simulink model "simulation"  (R2023b)
settings: Solver=ode1  StartTime=0.0  StopTime=90  FixedStep=0.01  RelTol=1e-3
undefined symbols (not defined in the file): A, B, C, dNx, dNy, dSx, dSy, g, kFD, kFT_N, kFT_S, Ki, kMD, kMDR_N, kMDR_S, Kx, m, w_hov, x0
libraries: SignalEditorBlockLib x1, shared6dof x1
settings Model: Creator=Rafa  LastModifiedBy=Rafa

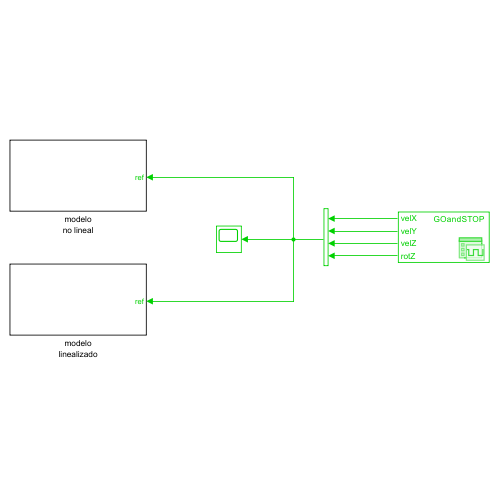
[thumbnail: Simulink's stored preview of the top-level diagram]
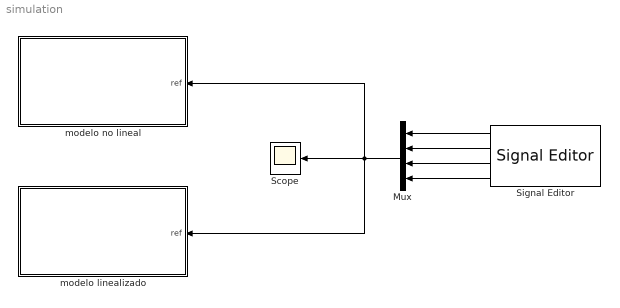
== system simulation ==
  Mux : Mux
  Scope : Scope
  Signal Editor : SignalEditorBlockLib/Signal Editor  FileName=C:\Users\Rafa\code\navsim\ws\src\navsim_pkg\models\UAM\aerotaxi\test\reference.mat  ActiveScenario=GOandSTOP  ActiveSignal=velX  IsBus=off  OutputBusObjectStr=Bus: BusObject  SampleTime=0  ZeroCross=off  OutputAfterFinalValue=Setting to zero  Unit=inherit  PreserveSignalName=on  ApplySigPropsToAllScenarios=on  ApplySigPropsToAllSignals=off
  modelo linealizado : Subsystem
      settings: PortSchema="{\"entries\":[{\"content\":{\"sides\":[{\"content\":{},\"type\":\"ConnectorPlacement.EquallySpacedRectSide\",\"uuid\":\"01253ba9-ebc4-4b01-a98e-e851f5719282\"},{\"content\":{\"connectorIds\":[\"In1\"],\"side\":\"RIGHT\"},\"type\":\"ConnectorPlacement.EquallySpacedRectSide\",\"uuid\":\"fb9dfd33-577f-4e16-aa58-2b7e19e1697c\"},{\"content\":{\"side\":\"TOP\"},\"type\":\"ConnectorPlacement.EquallySpacedRectSide\",\"uuid\":\"478e0daa-48f1-4d11-b0c5-5eb7f4b93804\"}]},\"type\":\"ConnectorPlacement.EquallySpacedConnector\",\"uuid\":\"8b8eac2c-ccef-432d-bf4d-f1cb8920e634\"}],\"packageUris\":[\"http://schema.mathworks.com/mf0/Connector/R2020b\"],\"version\":\"1.0\"}"
  modelo no lineal : Subsystem
      settings: PortSchema="{\"entries\":[{\"content\":{\"sides\":[{\"content\":{},\"type\":\"ConnectorPlacement.EquallySpacedRectSide\",\"uuid\":\"01253ba9-ebc4-4b01-a98e-e851f5719282\"},{\"content\":{\"connectorIds\":[\"In1\"],\"side\":\"RIGHT\"},\"type\":\"ConnectorPlacement.EquallySpacedRectSide\",\"uuid\":\"fb9dfd33-577f-4e16-aa58-2b7e19e1697c\"},{\"content\":{\"side\":\"TOP\"},\"type\":\"ConnectorPlacement.EquallySpacedRectSide\",\"uuid\":\"478e0daa-48f1-4d11-b0c5-5eb7f4b93804\"}]},\"type\":\"ConnectorPlacement.EquallySpacedConnector\",\"uuid\":\"8b8eac2c-ccef-432d-bf4d-f1cb8920e634\"}],\"packageUris\":[\"http://schema.mathworks.com/mf0/Connector/R2020b\"],\"version\":\"1.0\"}"
  wires:
  Signal Editor/4 -> Mux/4
  Signal Editor/2 -> Mux/2
  Signal Editor/1 -> Mux/1
  Signal Editor/3 -> Mux/3
  Mux/1 -> modelo linealizado/1(ref), modelo no lineal/1(ref), Scope/1

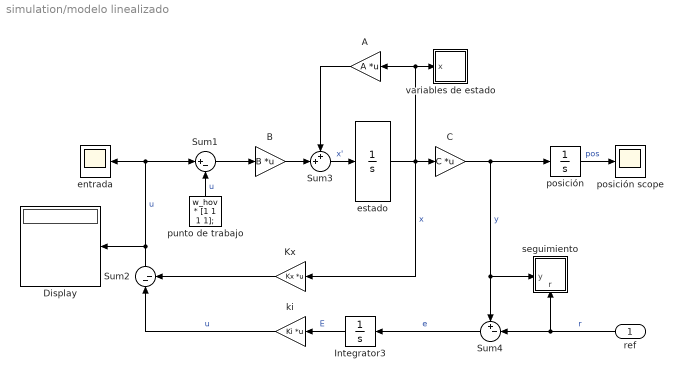
== system simulation/modelo linealizado ==
  ref : Inport
  A : Gain  Gain=A  Multiplication=Matrix(K*u)
  B : Gain  Gain=B  Multiplication=Matrix(K*u)
  C : Gain  Gain=C  Multiplication=Matrix(K*u)
  Display : Display
  Integrator3 : Integrator
  Kx : Gain  Gain=Kx  Multiplication=Matrix(K*u)
  Sum1 : Sum  Inputs=|+-
  Sum2 : Sum  Inputs=|--
  Sum3 : Sum  Inputs=++|
  Sum4 : Sum  Inputs=+-|
  entrada : Scope
  estado : Integrator  InitialCondition=x0
  ki : Gain  Gain=Ki  Multiplication=Matrix(K*u)
  posición : Integrator
  posición scope : Scope
  punto de trabajo : Constant  Value=w_hov * [1 1 1 1];
  seguimiento : Subsystem
      settings: PortSchema="{\"entries\":[{\"content\":{\"sides\":[{\"content\":{\"connectorIds\":[\"In1\"]},\"type\":\"ConnectorPlacement.EquallySpacedRectSide\",\"uuid\":\"d2eeeb7d-5f4a-4029-9315-eebcbcb452dd\"},{\"content\":{\"side\":\"RIGHT\"},\"type\":\"ConnectorPlacement.EquallySpacedRectSide\",\"uuid\":\"1640c7e1-69ae-41c3-aa10-8b2b7f223d3a\"},{\"content\":{\"side\":\"TOP\"},\"type\":\"ConnectorPlacement.EquallySpacedRectSide\",\"uuid\":\"4c9f5258-e874-4895-bd38-20065386e5c3\"},{\"content\":{\"connectorIds\":[\"In2\"],\"side\":\"BOTTOM\"},\"type\":\"ConnectorPlacement.EquallySpacedRectSide\",\"uuid\":\"545f1ef5-84f5-4856-98df-d523d3a0e9d2\"}]},\"type\":\"ConnectorPlacement.EquallySpacedConnector\",\"uuid\":\"43c46751-3b9a-4101-a1bf-f12efbef3486\"}],\"packageUris\":[\"http://schema.mathworks.com/mf0/Connector/R2020b\"],\"version\":\"1.0\"}"
  variables de estado : Subsystem
  wires:
  C/1 -> posición/1, Sum4/1, seguimiento/1(y)  "y"
  Sum1/1 -> B/1
  estado/1 -> Kx/1, A/1, variables de estado/1(x), C/1  "x"
  B/1 -> Sum3/2
  posición/1 -> posición scope/1  "pos"
  A/1 -> Sum3/1
  ref/1 -> seguimiento/2(r), Sum4/2  "r"
  ki/1 -> Sum2/1  "u"
  Sum4/1 -> Integrator3/1  "e"
  punto de trabajo/1 -> Sum1/2  "u"
  Sum2/1 -> Sum1/1, entrada/1, Display/1  "u"
  Sum3/1 -> estado/1  "x'"
  Kx/1 -> Sum2/2
  Integrator3/1 -> ki/1  "E"

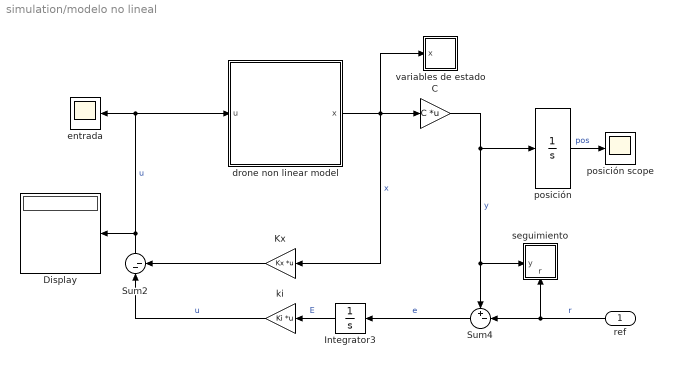
== system simulation/modelo no lineal ==
  ref : Inport
  C : Gain  Gain=C  Multiplication=Matrix(K*u)
  Display : Display
  Integrator3 : Integrator
  Kx : Gain  Gain=Kx  Multiplication=Matrix(K*u)
  Sum2 : Sum  Inputs=|--
  Sum4 : Sum  Inputs=+-|
  drone non linear model : Subsystem
  entrada : Scope
  ki : Gain  Gain=Ki  Multiplication=Matrix(K*u)
  posición : Integrator
  posición scope : Scope
  seguimiento : Subsystem
      settings: PortSchema="{\"entries\":[{\"content\":{\"sides\":[{\"content\":{\"connectorIds\":[\"In1\"]},\"type\":\"ConnectorPlacement.EquallySpacedRectSide\",\"uuid\":\"d2eeeb7d-5f4a-4029-9315-eebcbcb452dd\"},{\"content\":{\"side\":\"RIGHT\"},\"type\":\"ConnectorPlacement.EquallySpacedRectSide\",\"uuid\":\"1640c7e1-69ae-41c3-aa10-8b2b7f223d3a\"},{\"content\":{\"side\":\"TOP\"},\"type\":\"ConnectorPlacement.EquallySpacedRectSide\",\"uuid\":\"4c9f5258-e874-4895-bd38-20065386e5c3\"},{\"content\":{\"connectorIds\":[\"In2\"],\"side\":\"BOTTOM\"},\"type\":\"ConnectorPlacement.EquallySpacedRectSide\",\"uuid\":\"545f1ef5-84f5-4856-98df-d523d3a0e9d2\"}]},\"type\":\"ConnectorPlacement.EquallySpacedConnector\",\"uuid\":\"43c46751-3b9a-4101-a1bf-f12efbef3486\"}],\"packageUris\":[\"http://schema.mathworks.com/mf0/Connector/R2020b\"],\"version\":\"1.0\"}"
  variables de estado : Subsystem
  wires:
  Integrator3/1 -> ki/1  "E"
  Kx/1 -> Sum2/2
  Sum2/1 -> Display/1, drone non linear model/1(u), entrada/1  "u"
  Sum4/1 -> Integrator3/1  "e"
  ki/1 -> Sum2/1  "u"
  ref/1 -> Sum4/2, seguimiento/2(r)  "r"
  posición/1 -> posición scope/1  "pos"
  drone non linear model/1(x) -> C/1, variables de estado/1(x), Kx/1  "x"
  C/1 -> seguimiento/1(y), Sum4/1, posición/1  "y"

== system simulation/modelo linealizado/seguimiento ==
  y : Inport
  r : Inport  Port=2
  seguimiento de la referencia : Scope  NumInputPorts=2
  y Demux : Demux
  y Demux1 : Demux
  y Mux : Mux
  y Mux1 : Mux
  wires:
  y Demux/1 -> y Mux/1  "bXdot"
  y Demux/2 -> y Mux/2  "bYdot"
  y Demux/3 -> y Mux/3  "bZdot"
  y Mux/1 -> seguimiento de la referencia/1
  y Demux/4 -> y Mux/4  "bWz"
  y/1 -> y Demux/1
  r/1 -> y Demux1/1
  y Demux1/4 -> y Mux1/4  "bWz"
  y Mux1/1 -> seguimiento de la referencia/2
  y Demux1/3 -> y Mux1/3  "bZdot"
  y Demux1/2 -> y Mux1/2  "bYdot"
  y Demux1/1 -> y Mux1/1  "bXdot"

== system simulation/modelo linealizado/variables de estado ==
  x : Inport
  Demux : Demux  Outputs=8
  Mux : Mux  Inputs=8
  estado : Scope
  wires:
  Demux/6 -> Mux/6  "bXdot"
  Demux/7 -> Mux/7  "bYdot"
  Demux/8 -> Mux/8  "bZdot"
  Demux/2 -> Mux/2  "eTheta"
  Mux/1 -> estado/1
  Demux/4 -> Mux/4  "bWy"
  Demux/5 -> Mux/5  "bWz"
  Demux/1 -> Mux/1  "ePhi"
  Demux/3 -> Mux/3  "bWx"
  x/1 -> Demux/1

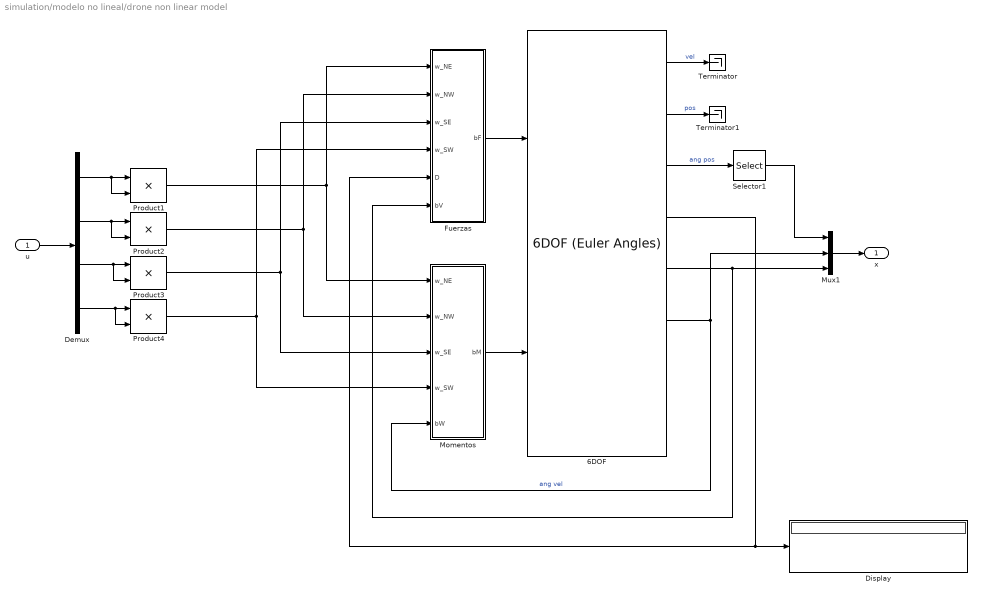
== system simulation/modelo no lineal/drone non linear model ==
  u : Inport
  6DOF : shared6dof/6DOF (Euler Angles)  units=Metric (MKS)  mtype=Fixed  rep=Euler Angles  xme_0=[0 0 0]  Vm_0=x0(6:8)  eul_0=[x0(1) x0(2) 0]  pm_0=x0(3:5)  mass_0=m  mass_e=0.5  mass_f=2.0  inertia=inertia  inertia_e=eye(3)  inertia_f=2*eye(3)  k_quat=1.0  vre_flag=on  abi_flag=off  aMode=aMode  xme_statename=''  Vm_statename=''  eul_statename=''  quat_statename=''  pm_statename=''  mass_statename=''
  Demux : Demux
  Display : Display
  Fuerzas : Subsystem
  Momentos : Subsystem
  Mux1 : Mux  Inputs=3
  Product{1..4} (4 alike) : Product
  Selector1 : Selector  InputPortWidth=3  IndexOptions=Index vector (dialog)  Indices=[1 2]  OutputSizes=1
  Terminator : Terminator
  Terminator1 : Terminator
  x : Outport  VectorParamsAs1DForOutWhenUnconnected=off
  wires:
  Product1/1 -> Fuerzas/1(w_NE), Momentos/1(w_NE)
  Product2/1 -> Fuerzas/2(w_NW), Momentos/2(w_NW)
  Product3/1 -> Fuerzas/3(w_SE), Momentos/3(w_SE)
  Product4/1 -> Fuerzas/4(w_SW), Momentos/4(w_SW)
  6DOF/4 -> Fuerzas/5(D), Display/1
  6DOF/6 -> Momentos/5(bW), Mux1/2  "ang vel"
  6DOF/5 -> Fuerzas/6(bV), Mux1/3
  6DOF/1 -> Terminator/1  "vel"
  6DOF/2 -> Terminator1/1  "pos"
  6DOF/3 -> Selector1/1  "ang pos"
  Mux1/1 -> x/1
  Selector1/1 -> Mux1/1
  u/1 -> Demux/1
  Fuerzas/1(bF) -> 6DOF/1
  Momentos/1(bM) -> 6DOF/2
  Demux/1 -> Product1/2, Product1/1
  Demux/2 -> Product2/2, Product2/1
  Demux/4 -> Product4/2, Product4/1
  Demux/3 -> Product3/2, Product3/1

== system simulation/modelo no lineal/seguimiento ==
  y : Inport
  r : Inport  Port=2
  seguimiento de la referencia : Scope  NumInputPorts=2
  y Demux : Demux
  y Demux1 : Demux
  y Mux : Mux
  y Mux1 : Mux
  wires:
  y Demux1/1 -> y Mux1/1  "bXdot"
  y Demux1/2 -> y Mux1/2  "bYdot"
  y Demux1/3 -> y Mux1/3  "bZdot"
  y Mux1/1 -> seguimiento de la referencia/2
  y Demux1/4 -> y Mux1/4  "bWz"
  r/1 -> y Demux1/1
  y/1 -> y Demux/1
  y Demux/4 -> y Mux/4  "bWz"
  y Mux/1 -> seguimiento de la referencia/1
  y Demux/3 -> y Mux/3  "bZdot"
  y Demux/2 -> y Mux/2  "bYdot"
  y Demux/1 -> y Mux/1  "bXdot"

== system simulation/modelo no lineal/variables de estado ==
  x : Inport
  Demux : Demux  Outputs=8
  Mux : Mux  Inputs=8
  estado : Scope
  wires:
  x/1 -> Demux/1
  Demux/3 -> Mux/3  "bWx"
  Demux/1 -> Mux/1  "ePhi"
  Demux/5 -> Mux/5  "bWz"
  Demux/4 -> Mux/4  "bWy"
  Mux/1 -> estado/1
  Demux/2 -> Mux/2  "eTheta"
  Demux/8 -> Mux/8  "bZdot"
  Demux/7 -> Mux/7  "bYdot"
  Demux/6 -> Mux/6  "bXdot"

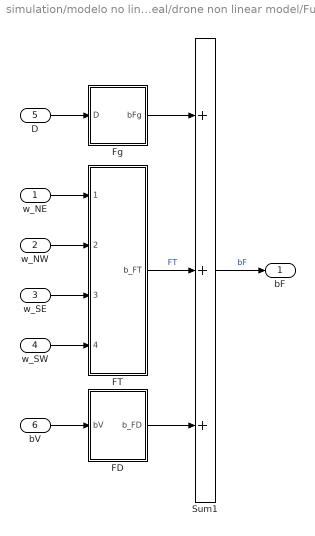
== system simulation/modelo no lineal/drone non linear model/Fuerzas ==
  w_NE : Inport
  w_NW : Inport  Port=2
  w_SE : Inport  Port=3
  w_SW : Inport  Port=4
  D : Inport  Port=5
  bV : Inport  Port=6
  FD : Subsystem
  FT : Subsystem
  Fg : Subsystem
  Sum1 : Sum  Inputs=+++
  bF : Outport  VectorParamsAs1DForOutWhenUnconnected=off
  wires:
  D/1 -> Fg/1(D)
  Fg/1(bFg) -> Sum1/1
  FT/1(b_FT) -> Sum1/2  "FT"
  w_SW/1 -> FT/4(w_SW)
  w_NE/1 -> FT/1(w_NE)
  w_SE/1 -> FT/3(w_SE)
  w_NW/1 -> FT/2(w_NW)
  Sum1/1 -> bF/1  "bF"
  bV/1 -> FD/1(bV)
  FD/1(b_FD) -> Sum1/3

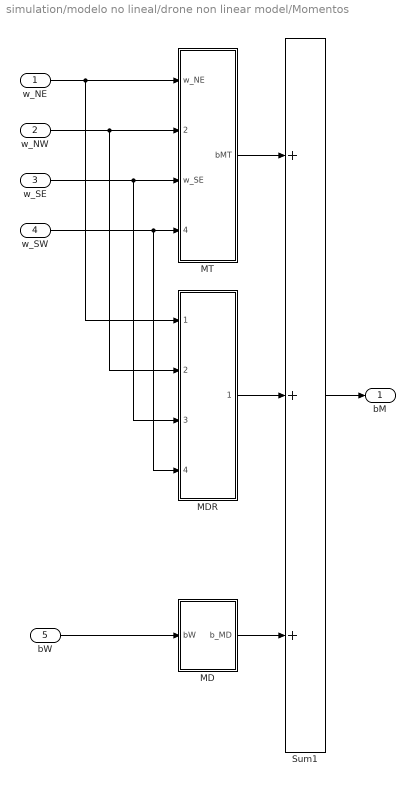
== system simulation/modelo no lineal/drone non linear model/Momentos ==
  w_NE : Inport
  w_NW : Inport  Port=2
  w_SE : Inport  Port=3
  w_SW : Inport  Port=4
  bW : Inport  Port=5
  MD : Subsystem
  MDR : Subsystem
  MT : Subsystem
  Sum1 : Sum  Inputs=+++
  bM : Outport  VectorParamsAs1DForOutWhenUnconnected=off
  wires:
  bW/1 -> MD/1(bW)
  MT/1(bMT) -> Sum1/1
  w_SW/1 -> MDR/4(w_SW), MT/4(w_SW)
  w_NE/1 -> MDR/1(w_NE), MT/1(w_NE)
  w_SE/1 -> MDR/3(w_SE), MT/3(w_SE)
  w_NW/1 -> MDR/2(w_NW), MT/2(w_NW)
  Sum1/1 -> bM/1
  MD/1(b_MD) -> Sum1/3
  MDR/1(b_MDR) -> Sum1/2

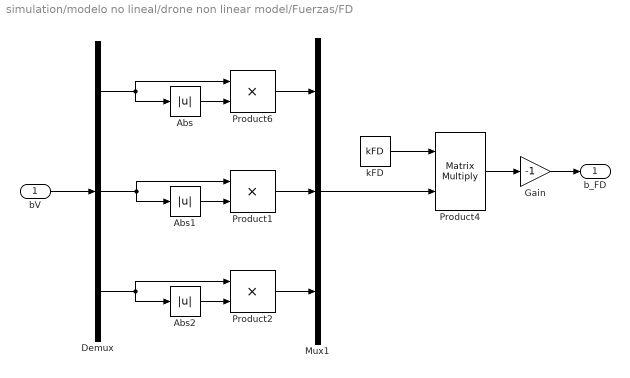
== system simulation/modelo no lineal/drone non linear model/Fuerzas/FD ==
  bV : Inport
  Abs : Abs  SaturateOnIntegerOverflow=off
  Abs1 : Abs  SaturateOnIntegerOverflow=off
  Abs2 : Abs  SaturateOnIntegerOverflow=off
  Demux : Demux  Outputs=3
  Gain : Gain  Gain=-1
  Mux1 : Mux  Inputs=3
  Product1 : Product
  Product2 : Product
  Product4 : Product  Multiplication=Matrix(*)
  Product6 : Product
  kFD : Constant  Value=kFD
  b_FD : Outport  VectorParamsAs1DForOutWhenUnconnected=off
  wires:
  kFD/1 -> Product4/1
  Product4/1 -> Gain/1
  Mux1/1 -> Product4/2
  Product1/1 -> Mux1/2
  bV/1 -> Demux/1
  Abs/1 -> Product6/2
  Abs1/1 -> Product1/2
  Abs2/1 -> Product2/2
  Demux/1 -> Product6/1, Abs/1
  Demux/2 -> Product1/1, Abs1/1
  Demux/3 -> Product2/1, Abs2/1
  Product6/1 -> Mux1/1
  Product2/1 -> Mux1/3
  Gain/1 -> b_FD/1

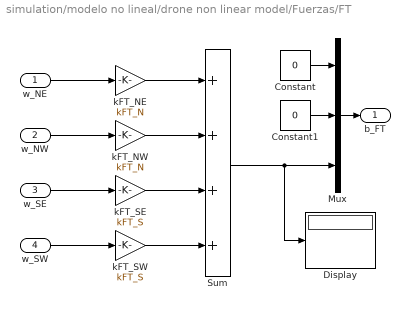
== system simulation/modelo no lineal/drone non linear model/Fuerzas/FT ==
  w_NE : Inport
  w_NW : Inport  Port=2
  w_SE : Inport  Port=3
  w_SW : Inport  Port=4
  Constant : Constant  Value=0
  Constant1 : Constant  Value=0
  Display : Display
  Mux : Mux  Inputs=3
  Sum : Sum  Inputs=++++
  kFT_NE : Gain  Gain=kFT_N
  kFT_NW : Gain  Gain=kFT_N
  kFT_SE : Gain  Gain=kFT_S
  kFT_SW : Gain  Gain=kFT_S
  b_FT : Outport  VectorParamsAs1DForOutWhenUnconnected=off
  wires:
  Mux/1 -> b_FT/1
  Constant/1 -> Mux/1
  Constant1/1 -> Mux/2
  Sum/1 -> Display/1, Mux/3
  w_NE/1 -> kFT_NE/1
  w_NW/1 -> kFT_NW/1
  w_SE/1 -> kFT_SE/1
  w_SW/1 -> kFT_SW/1
  kFT_NW/1 -> Sum/2
  kFT_NE/1 -> Sum/1
  kFT_SW/1 -> Sum/4
  kFT_SE/1 -> Sum/3

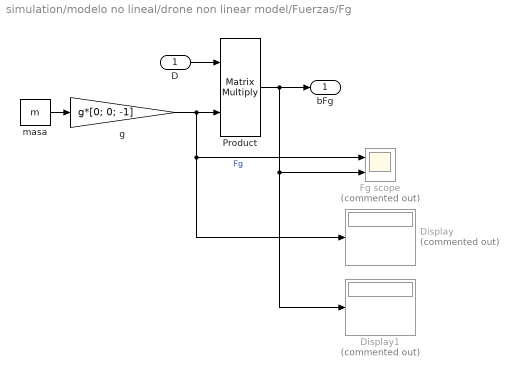
== system simulation/modelo no lineal/drone non linear model/Fuerzas/Fg ==
  D : Inport
  Display : Display  Commented=on
  Display1 : Display  Commented=on
  Fg scope : Scope  Commented=on  NumInputPorts=2
  Product : Product  Multiplication=Matrix(*)
  g : Gain  Gain=g*[0; 0; -1]
  masa : Constant  Value=m
  bFg : Outport  VectorParamsAs1DForOutWhenUnconnected=off
  wires:
  Product/1 -> Display1/1, Fg scope/2, bFg/1
  D/1 -> Product/1
  masa/1 -> g/1
  g/1 -> Display/1, Fg scope/1, Product/2  "Fg"

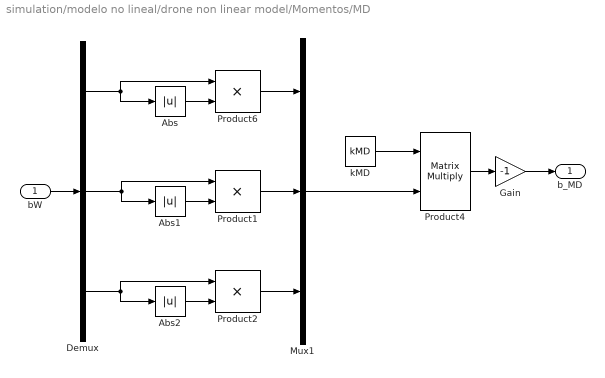
== system simulation/modelo no lineal/drone non linear model/Momentos/MD ==
  bW : Inport
  Abs : Abs  SaturateOnIntegerOverflow=off
  Abs1 : Abs  SaturateOnIntegerOverflow=off
  Abs2 : Abs  SaturateOnIntegerOverflow=off
  Demux : Demux  Outputs=3
  Gain : Gain  Gain=-1
  Mux1 : Mux  Inputs=3
  Product1 : Product
  Product2 : Product
  Product4 : Product  Multiplication=Matrix(*)
  Product6 : Product
  kMD : Constant  Value=kMD
  b_MD : Outport  VectorParamsAs1DForOutWhenUnconnected=off
  wires:
  kMD/1 -> Product4/1
  Product4/1 -> Gain/1
  Mux1/1 -> Product4/2
  Product1/1 -> Mux1/2
  bW/1 -> Demux/1
  Abs/1 -> Product6/2
  Abs1/1 -> Product1/2
  Abs2/1 -> Product2/2
  Demux/1 -> Product6/1, Abs/1
  Demux/2 -> Product1/1, Abs1/1
  Demux/3 -> Product2/1, Abs2/1
  Product6/1 -> Mux1/1
  Product2/1 -> Mux1/3
  Gain/1 -> b_MD/1

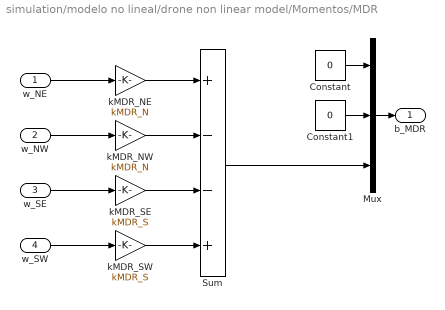
== system simulation/modelo no lineal/drone non linear model/Momentos/MDR ==
  w_NE : Inport
  w_NW : Inport  Port=2
  w_SE : Inport  Port=3
  w_SW : Inport  Port=4
  Constant : Constant  Value=0
  Constant1 : Constant  Value=0
  Mux : Mux  Inputs=3
  Sum : Sum  Inputs=+--+
  kMDR_NE : Gain  Gain=kMDR_N
  kMDR_NW : Gain  Gain=kMDR_N
  kMDR_SE : Gain  Gain=kMDR_S
  kMDR_SW : Gain  Gain=kMDR_S
  b_MDR : Outport  VectorParamsAs1DForOutWhenUnconnected=off
  wires:
  kMDR_SW/1 -> Sum/4
  kMDR_SE/1 -> Sum/3
  kMDR_NW/1 -> Sum/2
  kMDR_NE/1 -> Sum/1
  Mux/1 -> b_MDR/1
  Constant/1 -> Mux/1
  Constant1/1 -> Mux/2
  Sum/1 -> Mux/3
  w_SW/1 -> kMDR_SW/1
  w_SE/1 -> kMDR_SE/1
  w_NE/1 -> kMDR_NE/1
  w_NW/1 -> kMDR_NW/1

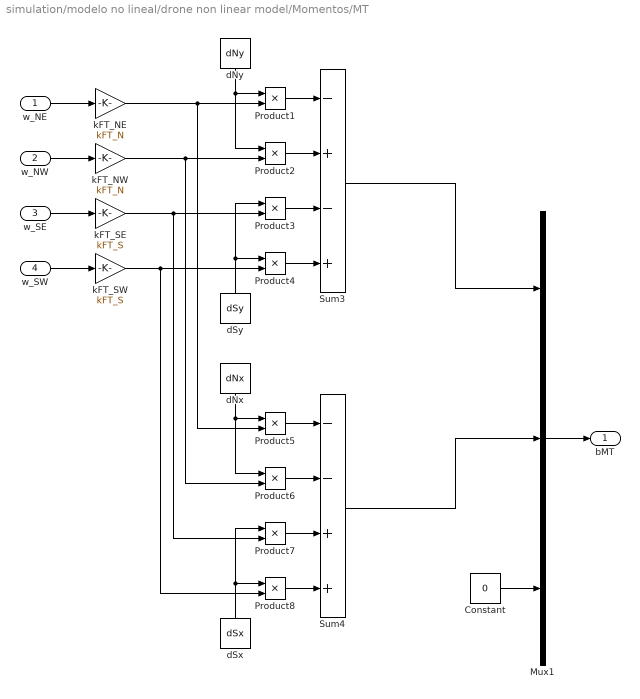
== system simulation/modelo no lineal/drone non linear model/Momentos/MT ==
  w_NE : Inport
  w_NW : Inport  Port=2
  w_SE : Inport  Port=3
  w_SW : Inport  Port=4
  Constant : Constant  Value=0
  Mux1 : Mux  Inputs=3
  Product{1..8} (8 alike) : Product
  Sum3 : Sum  Inputs=-+-+
  Sum4 : Sum  Inputs=--++
  dNx : Constant  Value=dNx
  dNy : Constant  Value=dNy
  dSx : Constant  Value=dSx
  dSy : Constant  Value=dSy
  kFT_NE : Gain  Gain=kFT_N
  kFT_NW : Gain  Gain=kFT_N
  kFT_SE : Gain  Gain=kFT_S
  kFT_SW : Gain  Gain=kFT_S
  bMT : Outport  VectorParamsAs1DForOutWhenUnconnected=off
  wires:
  Mux1/1 -> bMT/1
  Constant/1 -> Mux1/3
  kFT_NW/1 -> Product2/2, Product6/2
  kFT_NE/1 -> Product1/2, Product5/2
  kFT_SW/1 -> Product4/2, Product8/2
  w_NE/1 -> kFT_NE/1
  w_SE/1 -> kFT_SE/1
  kFT_SE/1 -> Product3/2, Product7/2
  w_NW/1 -> kFT_NW/1
  w_SW/1 -> kFT_SW/1
  Sum3/1 -> Mux1/1
  Sum4/1 -> Mux1/2
  dNy/1 -> Product1/1, Product2/1
  Product1/1 -> Sum3/1
  Product2/1 -> Sum3/2
  Product3/1 -> Sum3/3
  Product4/1 -> Sum3/4
  dSy/1 -> Product3/1, Product4/1
  Product5/1 -> Sum4/1
  Product6/1 -> Sum4/2
  Product7/1 -> Sum4/3
  Product8/1 -> Sum4/4
  dNx/1 -> Product6/1, Product5/1
  dSx/1 -> Product7/1, Product8/1
